simulink model "Problem3_AutomaticTransmissionControl"  (R2020b)
settings: Solver=ode5  StartTime=0.0  StopTime=50  FixedStep=0.04  RelTol=1e-3
PreLoadFcn:
  | clearvars
  | load('vehicleData.mat')
StartFcn:
  | cput= cputime;
StopFcn:
  | disp("CPU Time Elapsed"); cputime-cput
undefined symbols (not defined in the file): Iv, Kfactor, N20, Rfd, rload0, rload2, Rw, speedratio, Torkratio
CloseFcn:
  | clearvars
settings Model: DataDictionary=Data.sldd  Creator=vigne  LastModifiedBy=sushma

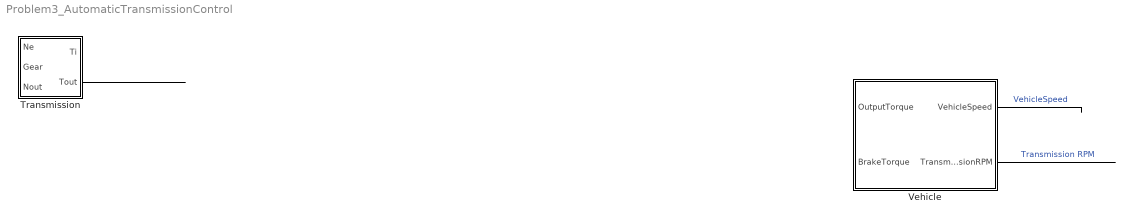
== system Problem3_AutomaticTransmissionControl ==
  Transmission : Subsystem
  Vehicle : Subsystem
  wires:
  Vehicle/2(TransmissionRPM) -> ?  "Transmission RPM"
  Vehicle/1(VehicleSpeed) -> ?  "VehicleSpeed"
  Transmission/2(Tout) -> ?

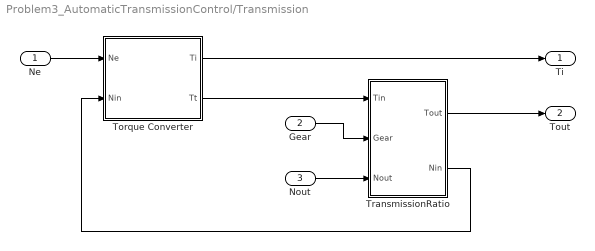
== system Problem3_AutomaticTransmissionControl/Transmission ==
  Ne : Inport  Unit=rpm
  Gear : Inport  Port=2  Unit=1
  Nout : Inport  Port=3  Unit=rpm
  Torque Converter : Subsystem
  TransmissionRatio : Subsystem
  Ti : Outport  Unit=ft*lbf@torque  VectorParamsAs1DForOutWhenUnconnected=off
  Tout : Outport  Port=2  Unit=ft*lbf@torque  VectorParamsAs1DForOutWhenUnconnected=off
  wires:
  Torque Converter/2(Tt) -> TransmissionRatio/1(Tin)
  Ne/1 -> Torque Converter/1(Ne)
  Torque Converter/1(Ti) -> Ti/1
  Nout/1 -> TransmissionRatio/3(Nout)
  Gear/1 -> TransmissionRatio/2(Gear)
  TransmissionRatio/2(Nin) -> Torque Converter/2(Nin)
  TransmissionRatio/1(Tout) -> Tout/1

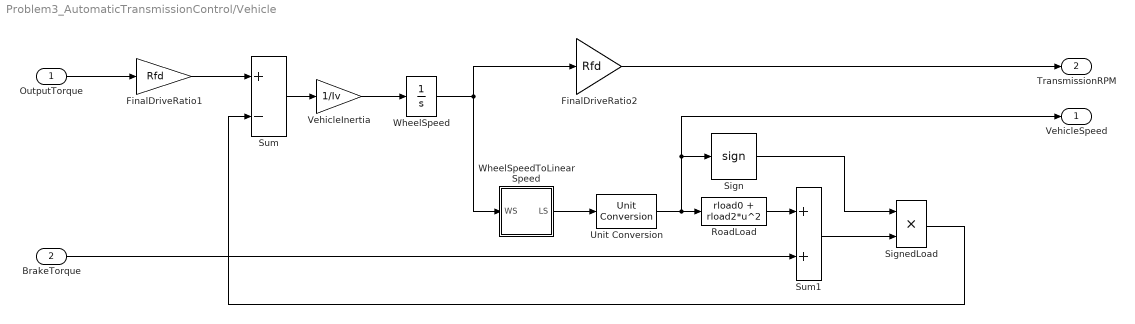
== system Problem3_AutomaticTransmissionControl/Vehicle ==
  OutputTorque : Inport  Unit=ft*lbf@torque
  BrakeTorque : Inport  Port=2  Unit=ft*lbf@torque
  FinalDriveRatio1 : Gain  Gain=Rfd  SaturateOnIntegerOverflow=on  OutDataTypeStr=Inherit: Same as input  ParamDataTypeStr=Inherit: Same as input
  FinalDriveRatio2 : Gain  Gain=Rfd  SaturateOnIntegerOverflow=on  OutDataTypeStr=Inherit: Same as input  ParamDataTypeStr=Inherit: Same as input
  RoadLoad : Fcn  Expr=rload0 + rload2*u^2
  Sign : Signum
  SignedLoad : Product  InputSameDT=on  SaturateOnIntegerOverflow=on  OutDataTypeStr=Inherit: Same as first input
  Sum : Sum  Inputs=+-  InputSameDT=on  SaturateOnIntegerOverflow=on  OutDataTypeStr=Inherit: Same as first input
  Sum1 : Sum  InputSameDT=on  SaturateOnIntegerOverflow=on  OutDataTypeStr=Inherit: Same as first input
  Unit Conversion : UnitConversion
  VehicleInertia : Gain  Gain=1/Iv  SaturateOnIntegerOverflow=on  OutDataTypeStr=Inherit: Same as input  ParamDataTypeStr=Inherit: Same as input
  WheelSpeed : Integrator  InitialCondition=N20/Rfd  ZeroCross=off
  WheelSpeedToLinearSpeed : Subsystem
  VehicleSpeed : Outport  Unit=mph  VectorParamsAs1DForOutWhenUnconnected=off
  TransmissionRPM : Outport  Port=2  Unit=rpm  VectorParamsAs1DForOutWhenUnconnected=off
  wires:
  FinalDriveRatio2/1 -> TransmissionRPM/1
  Unit Conversion/1 -> VehicleSpeed/1, Sign/1, RoadLoad/1
  OutputTorque/1 -> FinalDriveRatio1/1
  Sum1/1 -> SignedLoad/2
  WheelSpeed/1 -> FinalDriveRatio2/1, WheelSpeedToLinearSpeed/1(WS)
  WheelSpeedToLinearSpeed/1(LS) -> Unit Conversion/1
  Sum/1 -> VehicleInertia/1
  Sign/1 -> SignedLoad/1
  BrakeTorque/1 -> Sum1/2
  SignedLoad/1 -> Sum/2
  RoadLoad/1 -> Sum1/1
  VehicleInertia/1 -> WheelSpeed/1
  FinalDriveRatio1/1 -> Sum/1

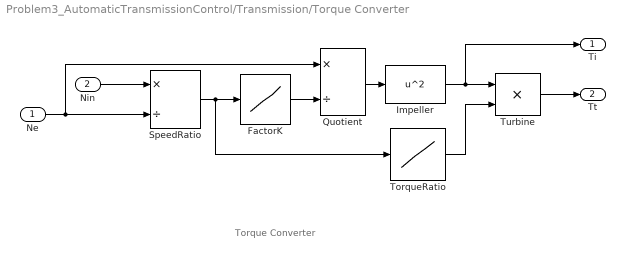
== system Problem3_AutomaticTransmissionControl/Transmission/Torque Converter ==
  note: Torque Converter
  Ne : Inport
  Nin : Inport  Port=2
  FactorK : Lookup_n-D  NumberOfTableDimensions=1  BreakpointsForDimension1=speedratio  Table=Kfactor  SaturateOnIntegerOverflow=on  InputSameDT=on
  Impeller : Fcn  Expr=u^2
  Quotient : Product  Inputs=*/  InputSameDT=on  SaturateOnIntegerOverflow=on  OutDataTypeStr=Inherit: Same as first input
  SpeedRatio : Product  Inputs=*/  InputSameDT=on  SaturateOnIntegerOverflow=on  OutDataTypeStr=Inherit: Same as first input
  TorqueRatio : Lookup_n-D  NumberOfTableDimensions=1  BreakpointsForDimension1=speedratio  Table=Torkratio  SaturateOnIntegerOverflow=on  InputSameDT=on
  Turbine : Product  InputSameDT=on  SaturateOnIntegerOverflow=on  OutDataTypeStr=Inherit: Same as first input
  Ti : Outport  VectorParamsAs1DForOutWhenUnconnected=off
  Tt : Outport  Port=2  VectorParamsAs1DForOutWhenUnconnected=off
  wires:
  Quotient/1 -> Impeller/1
  TorqueRatio/1 -> Turbine/2
  FactorK/1 -> Quotient/2
  Ne/1 -> SpeedRatio/2, Quotient/1
  Nin/1 -> SpeedRatio/1
  SpeedRatio/1 -> TorqueRatio/1, FactorK/1
  Impeller/1 -> Ti/1, Turbine/1
  Turbine/1 -> Tt/1

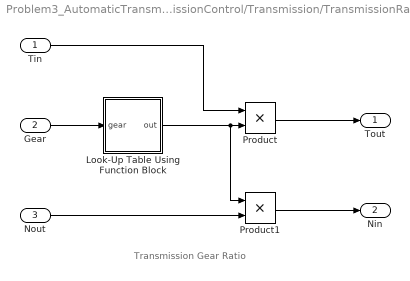
== system Problem3_AutomaticTransmissionControl/Transmission/TransmissionRatio ==
  note: Transmission Gear Ratio
  Tin : Inport  Unit=ft*lbf@torque
  Gear : Inport  Port=2  Unit=1
  Nout : Inport  Port=3  Unit=rpm
  Look-Up Table Using Function Block : MATLAB Function  TreatAsAtomicUnit=on
  Product : Product  InputSameDT=on  SaturateOnIntegerOverflow=on  OutDataTypeStr=Inherit: Same as first input
  Product1 : Product  InputSameDT=on  SaturateOnIntegerOverflow=on  OutDataTypeStr=Inherit: Same as first input
  Tout : Outport  Unit=ft*lbf@torque  VectorParamsAs1DForOutWhenUnconnected=off
  Nin : Outport  Port=2  Unit=rpm  VectorParamsAs1DForOutWhenUnconnected=off
  wires:
  Nout/1 -> Product1/2
  Look-Up Table Using Function Block/1(out) -> Product1/1, Product/2
  Product1/1 -> Nin/1
  Gear/1 -> Look-Up Table Using Function Block/1(gear)
  Tin/1 -> Product/1
  Product/1 -> Tout/1

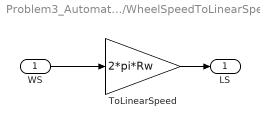
== system Problem3_AutomaticTransmissionControl/Vehicle/WheelSpeedToLinearSpeed ==
  WS : Inport  Unit=rpm
  ToLinearSpeed : Gain  Gain=2*pi*Rw  SaturateOnIntegerOverflow=on  OutDataTypeStr=Inherit: Same as input  ParamDataTypeStr=Inherit: Same as input
  LS : Outport  Unit=ft/min  VectorParamsAs1DForOutWhenUnconnected=off
  wires:
  ToLinearSpeed/1 -> LS/1
  WS/1 -> ToLinearSpeed/1

== matlab function Problem3_AutomaticTransmissionControl/Transmission/TransmissionRatio/Look-Up Table Using Function Block ==
  data: gear input; out output
function out = fcn(gear)
    %#codegen
    table = [2.393 1.450 1.000 0.677];
    switch(gear)
        case gearType.fourth;
            out=table(4);        
        case gearType.third;
            out=table(3);            
        case gearType.second;
            out=table(2);
        otherwise; % gearType.first
            out=table(1);
    end
    
end
